simulink model "ControleTrajNominalSimulink"  (R2019a)
settings: Solver=VariableStepAuto  StartTime=0.0  StopTime=170  RelTol=1e-3
undefined symbols (not defined in the file): A, B, C, D, K
settings Model: Creator=Cliente  LastModifiedBy=Cliente

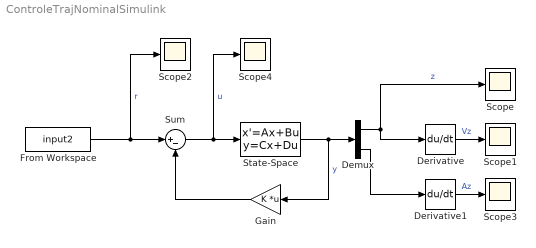
== system ControleTrajNominalSimulink ==
  Demux : Demux  Outputs=2
  Derivative : Derivative
  Derivative1 : Derivative
  From Workspace : FromWorkspace  VariableName=input2  SampleTime=0
  Gain : Gain  Gain=K  Multiplication=Matrix(K*u) (u vector)
  Scope{,1..4} (5 alike) : Scope
  State-Space : StateSpace  A=A  B=B  C=C  D=D  InitialCondition=[0; 0]
  Sum : Sum  Inputs=|+-
  wires:
  Demux/2 -> Derivative1/1
  Derivative1/1 -> Scope3/1  "Az"
  Demux/1 -> Scope/1, Derivative/1  "z"
  State-Space/1 -> Demux/1, Gain/1  "y"
  Derivative/1 -> Scope1/1  "Vz"
  Gain/1 -> Sum/2
  Sum/1 -> State-Space/1, Scope4/1  "u"
  From Workspace/1 -> Sum/1, Scope2/1  "r"
